simulink model "final_net_simout"  (Simulink 7.3)
settings: Solver=ode45  StartTime=0.0  StopTime=1  RelTol=1e-3
undefined symbols (not defined in the file): x
libraries: powerlib_extras x125, powerlib x91
(part 2 of 2)

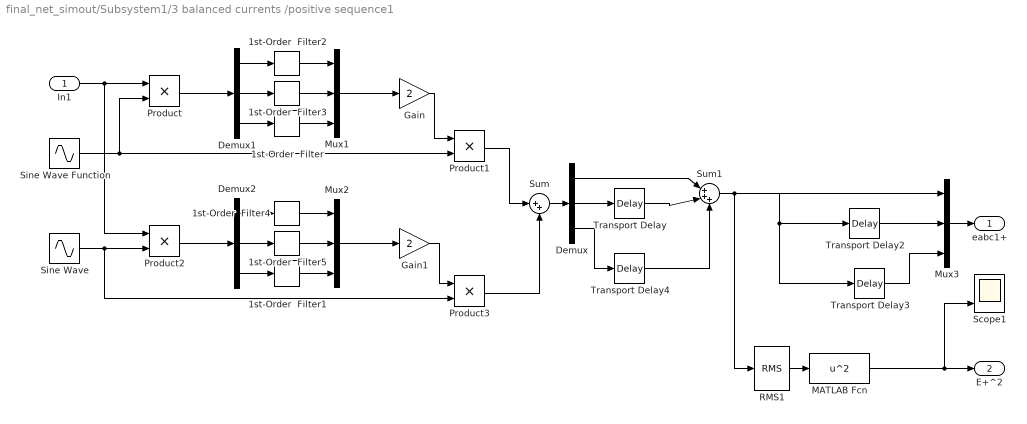
== system final_net_simout/Subsystem1/3 balanced currents /positive sequence1 ==
  In1 : Inport  OutDataType=sfix(16)  OutScaling=2^0
  1st-Order  Filter{,1,3,5} (4 alike) : powerlib_extras/Control  Blocks/1st-Order  Filter  DialogController=POWERSYS.PowerSysDialog  SystemSampleTime=-1  FilterType=Lowpass  Tc=.01  Initialize=off  Vac_Init=[0.8 -25 60]  Vdc_Init=-0.4  PlotResponse=off  param1=[1 500 1]
  1st-Order  Filter2 : powerlib_extras/Control  Blocks/1st-Order  Filter  DialogController=POWERSYS.PowerSysDialog  SystemSampleTime=-1  FilterType=Lowpass  Tc=.015  Initialize=off  Vac_Init=[0.8 -25 60]  Vdc_Init=-0.4  PlotResponse=off  param1=[1 500 1]
  1st-Order  Filter4 : powerlib_extras/Control  Blocks/1st-Order  Filter  DialogController=POWERSYS.PowerSysDialog  SystemSampleTime=-1  FilterType=Lowpass  Tc=.015  Initialize=off  Vac_Init=[0.8 -25 60]  Vdc_Init=-0.4  PlotResponse=off  param1=[1 500 1]
  Demux : Demux  Outputs=3
  Demux1 : Demux  Outputs=3
  Demux2 : Demux  Outputs=3
  Gain : Gain  Gain=2  ParameterDataType=sfix(16)  ParameterScaling=2^0  OutDataType=sfix(16)  OutScaling=2^0
  Gain1 : Gain  Gain=2  ParameterDataType=sfix(16)  ParameterScaling=2^0  OutDataType=sfix(16)  OutScaling=2^0
  MATLAB Fcn : MATLABFcn  MATLABFcn=u^2
  Mux1 : Mux  Inputs=3
  Mux2 : Mux  Inputs=3
  Mux3 : Mux  Inputs=3
  Product{,1..3} (4 alike) : Product  OutDataType=sfix(16)  OutScaling=2^0  RndMeth=Zero
  RMS1 : powerlib_extras/Measurements/RMS  DialogController=POWERSYS.PowerSysDialog  SystemSampleTime=-1  f1=50
  Scope1 : Scope  NumInputPorts=3
      settings: YMin=-1~-1~150000  YMax=1~1~320000
  Sine Wave : Sin  Amplitude=1  Bias=0  Frequency=100*pi  Phase=pi/2  Samples=10  SampleTime=0  Offset=0
  Sine Wave Function : Sin  Amplitude=1  Bias=0  Frequency=100*pi  Phase=0  Samples=10  SampleTime=0  Offset=0
  Sum : Sum  Inputs=|++  OutDataType=sfix(16)  OutScaling=2^0
  Sum1 : Sum  Inputs=|+++  OutDataType=sfix(16)  OutScaling=2^0
  Transport Delay : TransportDelay  DelayTime=.04/3
  Transport Delay2 : TransportDelay  DelayTime=.02/3
  Transport Delay3 : TransportDelay  DelayTime=.04/3
  Transport Delay4 : TransportDelay  DelayTime=.02/3
  eabc1+ : Outport  OutDataType=sfix(16)  OutScaling=2^0
  E+^2 : Outport  Port=2  OutDataType=sfix(16)  OutScaling=2^0
  wires:
  RMS1/1 -> MATLAB Fcn/1
  MATLAB Fcn/1 -> E+^2/1, Scope1/3
  In1/1 -> Product/1, Product2/1
  Sine Wave Function/1 -> Product/2, Product1/2
  1st-Order  Filter/1 -> Mux1/3
  Gain/1 -> Product1/1
  Sine Wave/1 -> Product2/2, Product3/2
  Gain1/1 -> Product3/1
  Product1/1 -> Sum/1
  Product3/1 -> Sum/2
  Sum/1 -> Demux/1
  Demux/2 -> Transport Delay/1
  Sum1/1 -> Transport Delay3/1, Mux3/1, RMS1/1, Transport Delay2/1
  Demux/3 -> Transport Delay4/1
  Transport Delay2/1 -> Mux3/2
  Transport Delay3/1 -> Mux3/3
  Mux3/1 -> eabc1+/1
  Demux1/1 -> 1st-Order  Filter2/1
  Demux1/2 -> 1st-Order  Filter3/1
  Demux1/3 -> 1st-Order  Filter/1
  Product/1 -> Demux1/1
  1st-Order  Filter2/1 -> Mux1/1
  1st-Order  Filter3/1 -> Mux1/2
  Mux1/1 -> Gain/1
  1st-Order  Filter1/1 -> Mux2/3
  Demux2/1 -> 1st-Order  Filter4/1
  Demux2/2 -> 1st-Order  Filter5/1
  Demux2/3 -> 1st-Order  Filter1/1
  Product2/1 -> Demux2/1
  1st-Order  Filter4/1 -> Mux2/1
  1st-Order  Filter5/1 -> Mux2/2
  Mux2/1 -> Gain1/1
  Demux/1 -> Sum1/1
  Transport Delay/1 -> Sum1/2
  Transport Delay4/1 -> Sum1/3

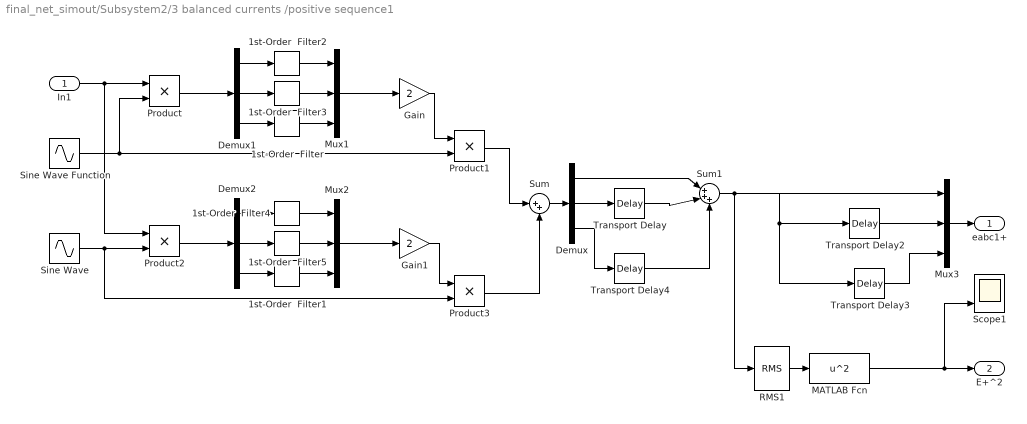
== system final_net_simout/Subsystem2/3 balanced currents /positive sequence1 ==
  In1 : Inport  OutDataType=sfix(16)  OutScaling=2^0
  1st-Order  Filter{,1,3,5} (4 alike) : powerlib_extras/Control  Blocks/1st-Order  Filter  DialogController=POWERSYS.PowerSysDialog  SystemSampleTime=-1  FilterType=Lowpass  Tc=.01  Initialize=off  Vac_Init=[0.8 -25 60]  Vdc_Init=-0.4  PlotResponse=off  param1=[1 500 1]
  1st-Order  Filter2 : powerlib_extras/Control  Blocks/1st-Order  Filter  DialogController=POWERSYS.PowerSysDialog  SystemSampleTime=-1  FilterType=Lowpass  Tc=.015  Initialize=off  Vac_Init=[0.8 -25 60]  Vdc_Init=-0.4  PlotResponse=off  param1=[1 500 1]
  1st-Order  Filter4 : powerlib_extras/Control  Blocks/1st-Order  Filter  DialogController=POWERSYS.PowerSysDialog  SystemSampleTime=-1  FilterType=Lowpass  Tc=.015  Initialize=off  Vac_Init=[0.8 -25 60]  Vdc_Init=-0.4  PlotResponse=off  param1=[1 500 1]
  Demux : Demux  Outputs=3
  Demux1 : Demux  Outputs=3
  Demux2 : Demux  Outputs=3
  Gain : Gain  Gain=2  ParameterDataType=sfix(16)  ParameterScaling=2^0  OutDataType=sfix(16)  OutScaling=2^0
  Gain1 : Gain  Gain=2  ParameterDataType=sfix(16)  ParameterScaling=2^0  OutDataType=sfix(16)  OutScaling=2^0
  MATLAB Fcn : MATLABFcn  MATLABFcn=u^2
  Mux1 : Mux  Inputs=3
  Mux2 : Mux  Inputs=3
  Mux3 : Mux  Inputs=3
  Product{,1..3} (4 alike) : Product  OutDataType=sfix(16)  OutScaling=2^0  RndMeth=Zero
  RMS1 : powerlib_extras/Measurements/RMS  DialogController=POWERSYS.PowerSysDialog  SystemSampleTime=-1  f1=50
  Scope1 : Scope  NumInputPorts=3
      settings: YMin=-1~-1~150000  YMax=1~1~320000
  Sine Wave : Sin  Amplitude=1  Bias=0  Frequency=100*pi  Phase=pi/2  Samples=10  SampleTime=0  Offset=0
  Sine Wave Function : Sin  Amplitude=1  Bias=0  Frequency=100*pi  Phase=0  Samples=10  SampleTime=0  Offset=0
  Sum : Sum  Inputs=|++  OutDataType=sfix(16)  OutScaling=2^0
  Sum1 : Sum  Inputs=|+++  OutDataType=sfix(16)  OutScaling=2^0
  Transport Delay : TransportDelay  DelayTime=.04/3
  Transport Delay2 : TransportDelay  DelayTime=.02/3
  Transport Delay3 : TransportDelay  DelayTime=.04/3
  Transport Delay4 : TransportDelay  DelayTime=.02/3
  eabc1+ : Outport  OutDataType=sfix(16)  OutScaling=2^0
  E+^2 : Outport  Port=2  OutDataType=sfix(16)  OutScaling=2^0
  wires:
  RMS1/1 -> MATLAB Fcn/1
  MATLAB Fcn/1 -> E+^2/1, Scope1/3
  In1/1 -> Product/1, Product2/1
  Sine Wave Function/1 -> Product/2, Product1/2
  1st-Order  Filter/1 -> Mux1/3
  Gain/1 -> Product1/1
  Sine Wave/1 -> Product2/2, Product3/2
  Gain1/1 -> Product3/1
  Product1/1 -> Sum/1
  Product3/1 -> Sum/2
  Sum/1 -> Demux/1
  Demux/2 -> Transport Delay/1
  Sum1/1 -> Transport Delay3/1, Mux3/1, RMS1/1, Transport Delay2/1
  Demux/3 -> Transport Delay4/1
  Transport Delay2/1 -> Mux3/2
  Transport Delay3/1 -> Mux3/3
  Mux3/1 -> eabc1+/1
  Demux1/1 -> 1st-Order  Filter2/1
  Demux1/2 -> 1st-Order  Filter3/1
  Demux1/3 -> 1st-Order  Filter/1
  Product/1 -> Demux1/1
  1st-Order  Filter2/1 -> Mux1/1
  1st-Order  Filter3/1 -> Mux1/2
  Mux1/1 -> Gain/1
  1st-Order  Filter1/1 -> Mux2/3
  Demux2/1 -> 1st-Order  Filter4/1
  Demux2/2 -> 1st-Order  Filter5/1
  Demux2/3 -> 1st-Order  Filter1/1
  Product2/1 -> Demux2/1
  1st-Order  Filter4/1 -> Mux2/1
  1st-Order  Filter5/1 -> Mux2/2
  Mux2/1 -> Gain1/1
  Demux/1 -> Sum1/1
  Transport Delay/1 -> Sum1/2
  Transport Delay4/1 -> Sum1/3

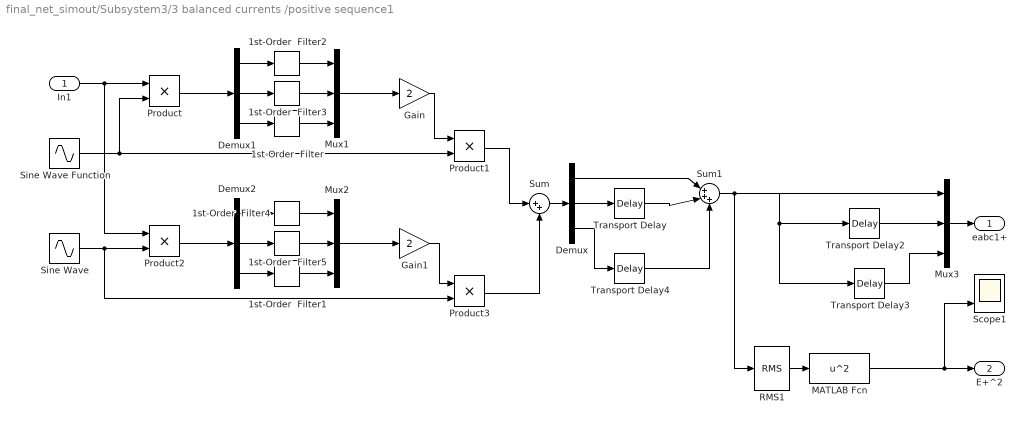
== system final_net_simout/Subsystem3/3 balanced currents /positive sequence1 ==
  In1 : Inport  OutDataType=sfix(16)  OutScaling=2^0
  1st-Order  Filter{,1,3,5} (4 alike) : powerlib_extras/Control  Blocks/1st-Order  Filter  DialogController=POWERSYS.PowerSysDialog  SystemSampleTime=-1  FilterType=Lowpass  Tc=.01  Initialize=off  Vac_Init=[0.8 -25 60]  Vdc_Init=-0.4  PlotResponse=off  param1=[1 500 1]
  1st-Order  Filter2 : powerlib_extras/Control  Blocks/1st-Order  Filter  DialogController=POWERSYS.PowerSysDialog  SystemSampleTime=-1  FilterType=Lowpass  Tc=.015  Initialize=off  Vac_Init=[0.8 -25 60]  Vdc_Init=-0.4  PlotResponse=off  param1=[1 500 1]
  1st-Order  Filter4 : powerlib_extras/Control  Blocks/1st-Order  Filter  DialogController=POWERSYS.PowerSysDialog  SystemSampleTime=-1  FilterType=Lowpass  Tc=.015  Initialize=off  Vac_Init=[0.8 -25 60]  Vdc_Init=-0.4  PlotResponse=off  param1=[1 500 1]
  Demux : Demux  Outputs=3
  Demux1 : Demux  Outputs=3
  Demux2 : Demux  Outputs=3
  Gain : Gain  Gain=2  ParameterDataType=sfix(16)  ParameterScaling=2^0  OutDataType=sfix(16)  OutScaling=2^0
  Gain1 : Gain  Gain=2  ParameterDataType=sfix(16)  ParameterScaling=2^0  OutDataType=sfix(16)  OutScaling=2^0
  MATLAB Fcn : MATLABFcn  MATLABFcn=u^2
  Mux1 : Mux  Inputs=3
  Mux2 : Mux  Inputs=3
  Mux3 : Mux  Inputs=3
  Product{,1..3} (4 alike) : Product  OutDataType=sfix(16)  OutScaling=2^0  RndMeth=Zero
  RMS1 : powerlib_extras/Measurements/RMS  DialogController=POWERSYS.PowerSysDialog  SystemSampleTime=-1  f1=50
  Scope1 : Scope  NumInputPorts=3
      settings: YMin=-1~-1~150000  YMax=1~1~320000
  Sine Wave : Sin  Amplitude=1  Bias=0  Frequency=100*pi  Phase=pi/2  Samples=10  SampleTime=0  Offset=0
  Sine Wave Function : Sin  Amplitude=1  Bias=0  Frequency=100*pi  Phase=0  Samples=10  SampleTime=0  Offset=0
  Sum : Sum  Inputs=|++  OutDataType=sfix(16)  OutScaling=2^0
  Sum1 : Sum  Inputs=|+++  OutDataType=sfix(16)  OutScaling=2^0
  Transport Delay : TransportDelay  DelayTime=.04/3
  Transport Delay2 : TransportDelay  DelayTime=.02/3
  Transport Delay3 : TransportDelay  DelayTime=.04/3
  Transport Delay4 : TransportDelay  DelayTime=.02/3
  eabc1+ : Outport  OutDataType=sfix(16)  OutScaling=2^0
  E+^2 : Outport  Port=2  OutDataType=sfix(16)  OutScaling=2^0
  wires:
  RMS1/1 -> MATLAB Fcn/1
  MATLAB Fcn/1 -> E+^2/1, Scope1/3
  In1/1 -> Product/1, Product2/1
  Sine Wave Function/1 -> Product/2, Product1/2
  1st-Order  Filter/1 -> Mux1/3
  Gain/1 -> Product1/1
  Sine Wave/1 -> Product2/2, Product3/2
  Gain1/1 -> Product3/1
  Product1/1 -> Sum/1
  Product3/1 -> Sum/2
  Sum/1 -> Demux/1
  Demux/2 -> Transport Delay/1
  Sum1/1 -> Transport Delay3/1, Mux3/1, RMS1/1, Transport Delay2/1
  Demux/3 -> Transport Delay4/1
  Transport Delay2/1 -> Mux3/2
  Transport Delay3/1 -> Mux3/3
  Mux3/1 -> eabc1+/1
  Demux1/1 -> 1st-Order  Filter2/1
  Demux1/2 -> 1st-Order  Filter3/1
  Demux1/3 -> 1st-Order  Filter/1
  Product/1 -> Demux1/1
  1st-Order  Filter2/1 -> Mux1/1
  1st-Order  Filter3/1 -> Mux1/2
  Mux1/1 -> Gain/1
  1st-Order  Filter1/1 -> Mux2/3
  Demux2/1 -> 1st-Order  Filter4/1
  Demux2/2 -> 1st-Order  Filter5/1
  Demux2/3 -> 1st-Order  Filter1/1
  Product2/1 -> Demux2/1
  1st-Order  Filter4/1 -> Mux2/1
  1st-Order  Filter5/1 -> Mux2/2
  Mux2/1 -> Gain1/1
  Demux/1 -> Sum1/1
  Transport Delay/1 -> Sum1/2
  Transport Delay4/1 -> Sum1/3

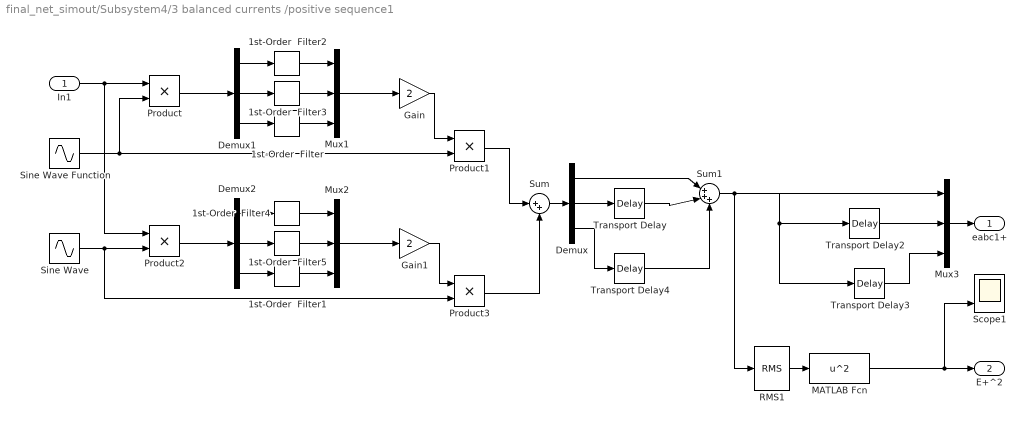
== system final_net_simout/Subsystem4/3 balanced currents /positive sequence1 ==
  In1 : Inport  OutDataType=sfix(16)  OutScaling=2^0
  1st-Order  Filter{,1,3,5} (4 alike) : powerlib_extras/Control  Blocks/1st-Order  Filter  DialogController=POWERSYS.PowerSysDialog  SystemSampleTime=-1  FilterType=Lowpass  Tc=.01  Initialize=off  Vac_Init=[0.8 -25 60]  Vdc_Init=-0.4  PlotResponse=off  param1=[1 500 1]
  1st-Order  Filter2 : powerlib_extras/Control  Blocks/1st-Order  Filter  DialogController=POWERSYS.PowerSysDialog  SystemSampleTime=-1  FilterType=Lowpass  Tc=.015  Initialize=off  Vac_Init=[0.8 -25 60]  Vdc_Init=-0.4  PlotResponse=off  param1=[1 500 1]
  1st-Order  Filter4 : powerlib_extras/Control  Blocks/1st-Order  Filter  DialogController=POWERSYS.PowerSysDialog  SystemSampleTime=-1  FilterType=Lowpass  Tc=.015  Initialize=off  Vac_Init=[0.8 -25 60]  Vdc_Init=-0.4  PlotResponse=off  param1=[1 500 1]
  Demux : Demux  Outputs=3
  Demux1 : Demux  Outputs=3
  Demux2 : Demux  Outputs=3
  Gain : Gain  Gain=2  ParameterDataType=sfix(16)  ParameterScaling=2^0  OutDataType=sfix(16)  OutScaling=2^0
  Gain1 : Gain  Gain=2  ParameterDataType=sfix(16)  ParameterScaling=2^0  OutDataType=sfix(16)  OutScaling=2^0
  MATLAB Fcn : MATLABFcn  MATLABFcn=u^2
  Mux1 : Mux  Inputs=3
  Mux2 : Mux  Inputs=3
  Mux3 : Mux  Inputs=3
  Product{,1..3} (4 alike) : Product  OutDataType=sfix(16)  OutScaling=2^0  RndMeth=Zero
  RMS1 : powerlib_extras/Measurements/RMS  DialogController=POWERSYS.PowerSysDialog  SystemSampleTime=-1  f1=50
  Scope1 : Scope  NumInputPorts=3
      settings: YMin=-1~-1~150000  YMax=1~1~320000
  Sine Wave : Sin  Amplitude=1  Bias=0  Frequency=100*pi  Phase=pi/2  Samples=10  SampleTime=0  Offset=0
  Sine Wave Function : Sin  Amplitude=1  Bias=0  Frequency=100*pi  Phase=0  Samples=10  SampleTime=0  Offset=0
  Sum : Sum  Inputs=|++  OutDataType=sfix(16)  OutScaling=2^0
  Sum1 : Sum  Inputs=|+++  OutDataType=sfix(16)  OutScaling=2^0
  Transport Delay : TransportDelay  DelayTime=.04/3
  Transport Delay2 : TransportDelay  DelayTime=.02/3
  Transport Delay3 : TransportDelay  DelayTime=.04/3
  Transport Delay4 : TransportDelay  DelayTime=.02/3
  eabc1+ : Outport  OutDataType=sfix(16)  OutScaling=2^0
  E+^2 : Outport  Port=2  OutDataType=sfix(16)  OutScaling=2^0
  wires:
  RMS1/1 -> MATLAB Fcn/1
  MATLAB Fcn/1 -> E+^2/1, Scope1/3
  In1/1 -> Product/1, Product2/1
  Sine Wave Function/1 -> Product/2, Product1/2
  1st-Order  Filter/1 -> Mux1/3
  Gain/1 -> Product1/1
  Sine Wave/1 -> Product2/2, Product3/2
  Gain1/1 -> Product3/1
  Product1/1 -> Sum/1
  Product3/1 -> Sum/2
  Sum/1 -> Demux/1
  Demux/2 -> Transport Delay/1
  Sum1/1 -> Transport Delay3/1, Mux3/1, RMS1/1, Transport Delay2/1
  Demux/3 -> Transport Delay4/1
  Transport Delay2/1 -> Mux3/2
  Transport Delay3/1 -> Mux3/3
  Mux3/1 -> eabc1+/1
  Demux1/1 -> 1st-Order  Filter2/1
  Demux1/2 -> 1st-Order  Filter3/1
  Demux1/3 -> 1st-Order  Filter/1
  Product/1 -> Demux1/1
  1st-Order  Filter2/1 -> Mux1/1
  1st-Order  Filter3/1 -> Mux1/2
  Mux1/1 -> Gain/1
  1st-Order  Filter1/1 -> Mux2/3
  Demux2/1 -> 1st-Order  Filter4/1
  Demux2/2 -> 1st-Order  Filter5/1
  Demux2/3 -> 1st-Order  Filter1/1
  Product2/1 -> Demux2/1
  1st-Order  Filter4/1 -> Mux2/1
  1st-Order  Filter5/1 -> Mux2/2
  Mux2/1 -> Gain1/1
  Demux/1 -> Sum1/1
  Transport Delay/1 -> Sum1/2
  Transport Delay4/1 -> Sum1/3
